simulink model "Currentreqtest"  (R2022a)
settings: Solver=FixedStepDiscrete  StartTime=0.0  StopTime=inf  FixedStep=0.01  RelTol=1e-3  EnableMultiTasking=on
libraries: mcp2515lib x32, simulink x29, svdutilitieslib x3, etargetslib x2
(part 1 of 2)
settings Model: Creator=Student  LastModifiedBy=Student
settings SolverCC: PositivePriorityOrder=on
settings OptimizationCC: EnhancedBackFolding=on  PassReuseOutputArgsAs=Individual arguments  ZeroExternalMemoryAtStartup=off  ZeroInternalMemoryAtStartup=off  MaxStackSize=64  OptimizeBlockOrder=speed  DifferentSizesBufferReuse=on  OptimizationCustomize=off  EfficientTunableParamExpr=on
settings DebuggingCC: ParameterTunabilityLossMsg=error
settings HardwareCC: ProdBitPerPointer=32  ProdBitPerSizeT=32  ProdBitPerPtrDiffT=32  ProdLargestAtomicInteger=Long  ProdLargestAtomicFloat=Double  ProdWordSize=32  ProdLongLongMode=on  ProdHWDeviceType=ARM Compatible->ARM Cortex  UseEmbeddedCoderFeatures=off
settings RTWCC: SystemTargetFile=ert.tlc  HardwareBoard=Raspberry Pi  TLCOptions="-aInlineSetEventsForThisBaseRateFcn=TLC_FALSE -aSuppressMultiTaskScheduler=TLC_FALSE  -aRateBasedStepFcn=0"  TemplateMakefile=ert_default_tmf  Toolchain=GNU GCC Embedded Linux  BuildConfiguration=Faster Runs
settings CodeAppCC: ForceParamTrailComments=on  IgnoreCustomStorageClasses=off  OperatorAnnotations=on  SimulinkDataObjDesc=on  SFDataObjDesc=on  InsertBlockDesc=on
settings ERTTargetCC: SupportNonInlinedSFcns=on  SupportVariableSizeSignals=on  ExtModeTransport=2  ExtModeStaticAlloc=on  ExtModeMexFile=ext_xcp  ExtModeIntrfLevel=Level2 - Open

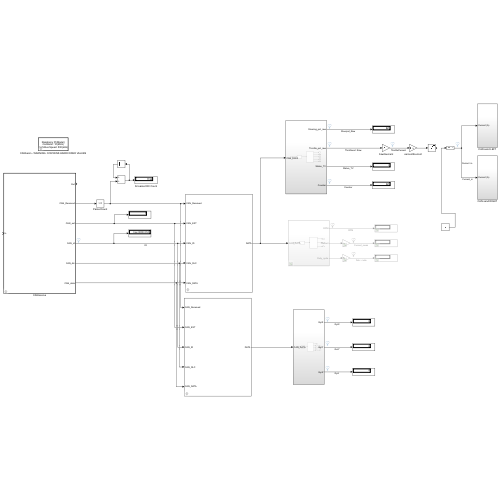
[thumbnail: Simulink's stored preview of the top-level diagram]
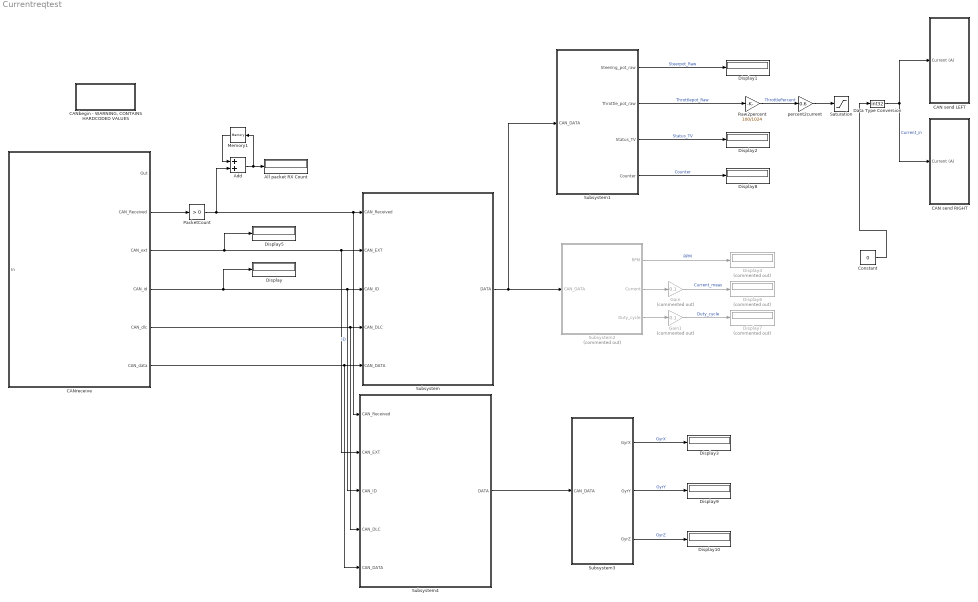
== system Currentreqtest ==
  Add : Sum  OutDataTypeStr=uint32
  All packet RX Count : Display
  CAN send LEFT : Subsystem
  CAN send RIGHT : Subsystem
  "CANbegin - WARNING, CONTAINS HARDCODED VALUES" : Subsystem  TreatAsAtomicUnit=on  mask{TargetHardware=Raspberry Pi, Oscillator=10, CANSpeed=500, CSpin=10}
      mask prompts: TargetHardware "Target Hardware"; Oscillator "Oscillator frequency(MHz)"; CANSpeed "CAN speed(kHz)"; CSpin "Chip Select Pin"
      mask init:
      | % Get this mask's handle
      | maskObj = Simulink.Mask.get(gcb);
      | 
      | % Get the selected value from mask parameter's option
      | str_TargetHard = char(maskObj.Parameters(1).TypeOptions(TargetHardware));
      | str_Osc = char(maskObj.Parameters(2).TypeOptions(Oscillator));
      | str_CANSpeed = char(maskObj.Parameters(3).TypeOptions(CANSpeed));
      | 
      | % Set Icon
      | str1 = sprintf('%s(Model)',str_TargetHard);
      | str2 = sprintf('Oscillator: %s(MHz)',str_Osc);
      | str3 = sprintf('CAN Bus Speed: %s(kHz)',str_CANSpeed);
      | str4 = sprintf('Chip Select pin: %d',CSpin);
      | 
      | % Set the values of Variant Subsystem
      | switch str_TargetHard
      |     case 'Arduino'
      |         str = [str1,'\n',str2,'\n',str3,'\n',str4];
      |         evalin('base',sprintf('CSpin = %d;',CSpin));        
      |         evalin('base','Hardware = 1;');
      |     case 'Raspberry Pi'
      |         str = [str1,'\n',str2,'\n',str3];
      |         evalin('base',sprintf('clear CSpin',CSpin));           
      |         evalin('base','Hardware = 2;');     
      | end  
      | 
      | % Get the CAN Configuration register's value from mask parameter's option
      | if str_Osc == '8' %[MHz]
      |     switch str_CANSpeed
      |         case '1000'
      |             BPR = 0; PHSEG1 = 0; PRSEG = 0; PHSEG2 = 0;
      |         case '500'
      |             BPR = 0; PHSEG1 = 2; PRSEG = 0; PHSEG2 = 2;
      |         case '250'
      |             BPR = 0; PHSEG1 = 6; PRSEG = 0; PHSEG2 = 6;
      |         case '125'
      |             BPR = 1; PHSEG1 = 6; PRSEG = 1; PHSEG2 = 5;
      |         case '100'
      |             BPR = 1; PHSEG1 = 7; PRSEG = 2; PHSEG2 = 7;
      |         case '83.3'
      |             BPR = 1; PHSEG1 = 7; PRSEG = 6; PHSEG2 = 7;
      |         case '62.5'
      |             BPR = 3; PHSEG1 = 6; PRSEG = 0; PHSEG2 = 6;
      |         case '50'
      |             BPR = 3; PHSEG1 = 7; PRSEG = 2; PHSEG2 = 7;
      |         case '33.3'
      |             BPR = 4; PHSEG1 = 7; PRSEG = 6; PHSEG2 = 7;
      |     end            
      | elseif str_Osc == '16' %[MHz]
      |     switch str_CANSpeed  
      |         case '1000'
      |             BPR = 0; PHSEG1 = 2; PRSEG = 0; PHSEG2 = 2;
      |         case '500'
      |             BPR = 0; PHSEG1 = 6; PRSEG = 0; PHSEG2 = 6;
      |         case '250'
      |             BPR = 1; PHSEG1 = 6; PRSEG = 1; PHSEG2 = 5;        
      |         case '125'
      |             BPR = 3; PHSEG1 = 6; PRSEG = 0; PHSEG2 = 6;
      |         case '100'
      |             BPR = 3; PHSEG1 = 7; PRSEG = 2; PHSEG2 = 7;
      |         case '83.3'
      |             BPR = 3; PHSEG1 = 7; PRSEG = 6; PHSEG2 = 7;
      |         case '62.5'
      |             BPR = 7; PHSEG1 = 6; PRSEG = 0; PHSEG2 = 6;
      |         case '50'
      |             BPR = 7; PHSEG1 = 7; PRSEG = 2; PHSEG2 = 7;
      |         case '33.3'
      |             BPR = 9; PHSEG1 = 7; PRSEG = 6; PHSEG2 = 7;        
      |     end
      |     
      | elseif str_Osc == '10' %[MHz]
      |     switch str_CANSpeed  
      |         case '1000'
      |             BPR = 0; PHSEG1 = 2; PRSEG = 0; PHSEG2 = 2;
      |         case '500'
      |             BPR = 0; PHSEG1 = 5; PRSEG = 0; PHSEG2 = 4;
      |         case '250'
      |             BPR = 1; PHSEG1 = 6; PRSEG = 1; PHSEG2 = 5;        
      |         case '125'
      |             BPR = 3; PHSEG1 = 6; PRSEG = 0; PHSEG2 = 6;
      |         case '100'
      |             BPR = 3; PHSEG1 = 7; PRSEG = 2; PHSEG2 = 7;
      |         case '83.3'
      |             BPR = 3; PHSEG1 = 7; PRSEG = 6; PHSEG2 = 7;
      |         case '62.5'
      |             BPR = 7; PHSEG1 = 6; PRSEG = 0; PHSEG2 = 6;
      |         case '50'
      |             BPR = 7; PHSEG1 = 7; PRSEG = 2; PHSEG2 = 7;
      |         case '33.3'
      |             BPR = 9; PHSEG1 = 7; PRSEG = 6; PHSEG2 = 7;        
      |     end    
      |     
      |     
      | end
      | % % Set the CAN Configuration register's value
      | % address2A = BPR;          % bit7-6 :SJW, bit5-0: BPR
      | % address29 = 192 ...       % bit7: BTLMODE = 1, bit6:SAM = 1
      | %             + 8*PHSEG1 ...% bit5-3: PHSEG1
      | %             +PRSEG;       % bit2-0: PRSEG
      | % address28 = 128 ...       % bit7: SOF = 1, bit6:WAKFIL = 0
      | %             + PHSEG2;     % bit5-3: 0, bit2-0: PHSEG2
      |         
      | % force parameters... 
      | % %1M CAN
      | % address2A=hex2dec('40')
      | % address29=hex2dec('80')
      | % address28=hex2dec('1')
      | 
      | %500k CAN
      | address2A=hex2dec('0')
      | address29=hex2dec('A0')
      | address28=hex2dec('02')
      | 
      | % %500k CAN from Arduino library spreadsheet - doesn't work
      | % address2A=hex2dec('41')
      | % address29=hex2dec('D9')
      | % address28=hex2dec('82')
      settings: RTWSystemCode=Nonreusable function
      mask TypeOptions TargetHardware: Arduino | Raspberry Pi
      mask Callback TargetHardware:
      | if(strcmp(get_param(gcb,'TargetHardware'),'Arduino'))
      |     set_param(gcb,'MaskVisibilities',{'on','on','on','on'})
      | else
      |     set_param(gcb,'MaskVisibilities',{'on','on','on','off'})
      | end
      mask TypeOptions Oscillator: 8 | 16 | 10
      mask TypeOptions CANSpeed: 1000 | 500 | 250 | 125 | 100 | 83.3 | 62.5 | 50 | 33.3
      mask DialogControl DescGroupVar Prompt: Description
      mask DialogControl DescTextVar Prompt: Forced parameters for 10MHz oscillator, 500k CAN This block must be executed only once when beginning CAN communication because MCP2515’s register needs to be configured. And the frequency of oscillator for MCP2515 is also needed because it effects to the setting parameters of MCP2515's register.
      mask Display: disp(str)
  CANreceive : Subsystem  TreatAsAtomicUnit=on
      mask DialogControl DescGroupVar Prompt: Description
      mask DialogControl DescTextVar Prompt: CANreceive outputs CAN data by converting MCP2515 RX buffer register’s values. In/Out ports are no use because they are used for controlling the execution order. CAN_Received outputs 1(CAN received) or -1( No message).
  Constant : Constant  Value=0
  Data Type Conversion : DataTypeConversion  OutDataTypeStr=int32  SaturateOnIntegerOverflow=off  RndMeth=Floor
  Display{,1..3,5,8..10} (8 alike) : Display
      Display settings: Format=hex (Stored Integer)
  Display4 : Display  Commented=on
  Display6 : Display  Commented=on
  Display7 : Display  Commented=on
  Gain : Gain  Commented=on  Gain=0.1
  Gain1 : Gain  Commented=on  Gain=0.1
  Memory1 : Memory  InitialCondition=[0]
  "PacketCount " : simulink/Logic and Bit Operations/Compare To Constant  relop=>  const=0  OutDataTypeStr=uint8
  Raw2percent : Gain  Gain=100/1024
  Saturation : Saturate  UpperLimit=40  LowerLimit=0
  Subsystem : Subsystem  mask{ID=0x123, DLC=6, EXT=1}
      mask prompts: ID "Message ID"; DLC "Message DLC"; EXT "Type of ID (1 is extended, 0 is standard)"
      mask DialogControl DescGroupVar Prompt: Filter CAN Data
      mask DialogControl DescTextVar Prompt: Give the ID and DLC of the CAN Message you want to get the data from
  Subsystem1 : Subsystem
  Subsystem2 : Subsystem  Commented=on
  Subsystem3 : Subsystem
  Subsystem4 : Subsystem  mask{ID=0x32, DLC=6, EXT=1}
      mask prompts: ID "Message ID"; DLC "Message DLC"; EXT "Type of ID (1 is extended, 0 is standard)"
      mask DialogControl DescGroupVar Prompt: Filter CAN Data
      mask DialogControl DescTextVar Prompt: Give the ID and DLC of the CAN Message you want to get the data from
  percent2current : Gain  Gain=0.6
  wires:
  Gain1/1 -> Display7/1  "Duty_cycle"
  "PacketCount "/1 -> Add/2, Subsystem4/1(CAN_Received), Subsystem/1(CAN_Received)
  Memory1/1 -> Add/1
  Subsystem2/3(Duty_cycle) -> Gain1/1
  Gain/1 -> Display6/1  "Current_meas"
  Subsystem2/1(RPM) -> Display4/1  "RPM"
  Subsystem1/1(Steering_pot_raw) -> Display1/1  "Steerpot_Raw"
  CANreceive/5(CAN_dlc) -> Subsystem/4(CAN_DLC), Subsystem4/4(CAN_DLC)
  Subsystem2/2(Current) -> Gain/1
  Subsystem1/3(Status_TV) -> Display2/1  "Status_TV"
  Subsystem1/2(Throttle_pot_raw) -> Raw2percent/1  "Throttlepot_Raw"
  CANreceive/4(CAN_id) -> Display/1, Subsystem/3(CAN_ID), Subsystem4/3(CAN_ID)  "ID"
  Add/1 -> All packet RX Count/1, Memory1/1
  Subsystem/1(DATA) -> Subsystem1/1(CAN_DATA), Subsystem2/1(CAN_DATA)
  CANreceive/3(CAN_ext) -> Display5/1, Subsystem/2(CAN_EXT), Subsystem4/2(CAN_EXT)
  CANreceive/2(CAN_Received) -> "PacketCount "/1
  CANreceive/6(CAN_data) -> Subsystem/5(CAN_DATA), Subsystem4/5(CAN_DATA)
  Data Type Conversion/1 -> CAN send RIGHT/1(Current (A)), CAN send LEFT/1(Current (A))  "Current_in"
  Subsystem1/4(Counter) -> Display8/1  "Counter"
  Raw2percent/1 -> percent2current/1  "ThrottlePercent"
  percent2current/1 -> Saturation/1
  Subsystem3/1(GyrX) -> Display3/1  "GyrX"
  Subsystem3/2(GyrY) -> Display9/1  "GyrY"
  Subsystem3/3(GyrZ) -> Display10/1  "GyrZ"
  Subsystem4/1(DATA) -> Subsystem3/1(CAN_DATA)
  Constant/1 -> Data Type Conversion/1

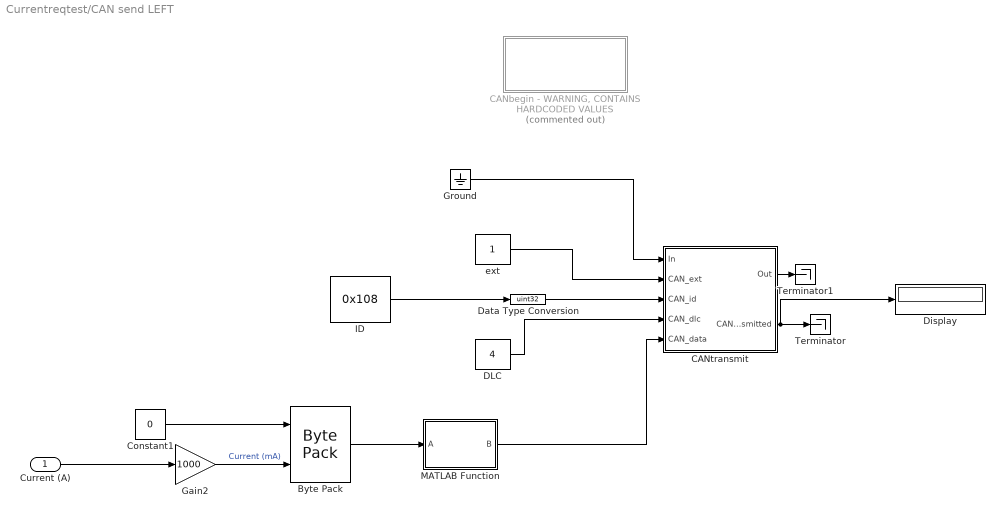
== system Currentreqtest/CAN send LEFT ==
  Current (A) : Inport  OutDataTypeStr=int32
  Byte Pack : etargetslib/Byte Pack  datatypes={'int32','int32'}  byteAlign=1
  "CANbegin - WARNING, CONTAINS HARDCODED VALUES" : Subsystem  Commented=on  TreatAsAtomicUnit=on  mask{TargetHardware=Raspberry Pi, Oscillator=10, CANSpeed=500, CSpin=10}
      mask prompts: TargetHardware "Target Hardware"; Oscillator "Oscillator frequency(MHz)"; CANSpeed "CAN speed(kHz)"; CSpin "Chip Select Pin"
      mask init: same as Currentreqtest/CANbegin - WARNING, CONTAINS HARDCODED VALUES
      settings: RTWSystemCode=Nonreusable function
      mask TypeOptions TargetHardware: Arduino | Raspberry Pi
      mask Callback TargetHardware:
      | if(strcmp(get_param(gcb,'TargetHardware'),'Arduino'))
      |     set_param(gcb,'MaskVisibilities',{'on','on','on','on'})
      | else
      |     set_param(gcb,'MaskVisibilities',{'on','on','on','off'})
      | end
      mask TypeOptions Oscillator: 8 | 16 | 10
      mask TypeOptions CANSpeed: 1000 | 500 | 250 | 125 | 100 | 83.3 | 62.5 | 50 | 33.3
      mask DialogControl DescGroupVar Prompt: Description
      mask DialogControl DescTextVar Prompt: Forced parameters for 10MHz oscillator, 500k CAN This block must be executed only once when beginning CAN communication because MCP2515’s register needs to be configured. And the frequency of oscillator for MCP2515 is also needed because it effects to the setting parameters of MCP2515's register.
      mask Display: disp(str)
  CANtransmit : Subsystem  TreatAsAtomicUnit=on
      mask DialogControl DescGroupVar Prompt: Description
      mask DialogControl DescTextVar Prompt: CANtransmit inputs CAN data by converting MCP2515 TX buffer register’s values. In/Out ports are no use because they are used for controlling the execution order. CAN_Transmitted outputs 1(Success) or 2(Fail).
  Constant1 : Constant  Value=0  OutDataTypeStr=int32
  DLC : Constant  Value=4  OutDataTypeStr=uint8
  Data Type Conversion : DataTypeConversion  OutDataTypeStr=uint32  SaturateOnIntegerOverflow=off  RndMeth=Floor
  Display : Display
  Gain2 : Gain  Gain=1000  OutDataTypeStr=int32
  Ground : Ground
  ID : Constant  Value=0x108  OutDataTypeStr=uint32
  MATLAB Function : MATLAB Function  TreatAsAtomicUnit=on
  Terminator : Terminator
  Terminator1 : Terminator
  ext : Constant  OutDataTypeStr=uint8
  wires:
  Byte Pack/1 -> MATLAB Function/1(A)
  Ground/1 -> CANtransmit/1(In)
  ext/1 -> CANtransmit/2(CAN_ext)
  DLC/1 -> CANtransmit/4(CAN_dlc)
  CANtransmit/1(Out) -> Terminator1/1
  CANtransmit/2(CAN_Transmitted) -> Display/1, Terminator/1
  Data Type Conversion/1 -> CANtransmit/3(CAN_id)
  Constant1/1 -> Byte Pack/1
  MATLAB Function/1(B) -> CANtransmit/5(CAN_data)
  Current (A)/1 -> Gain2/1
  Gain2/1 -> Byte Pack/2  "Current (mA)"
  ID/1 -> Data Type Conversion/1

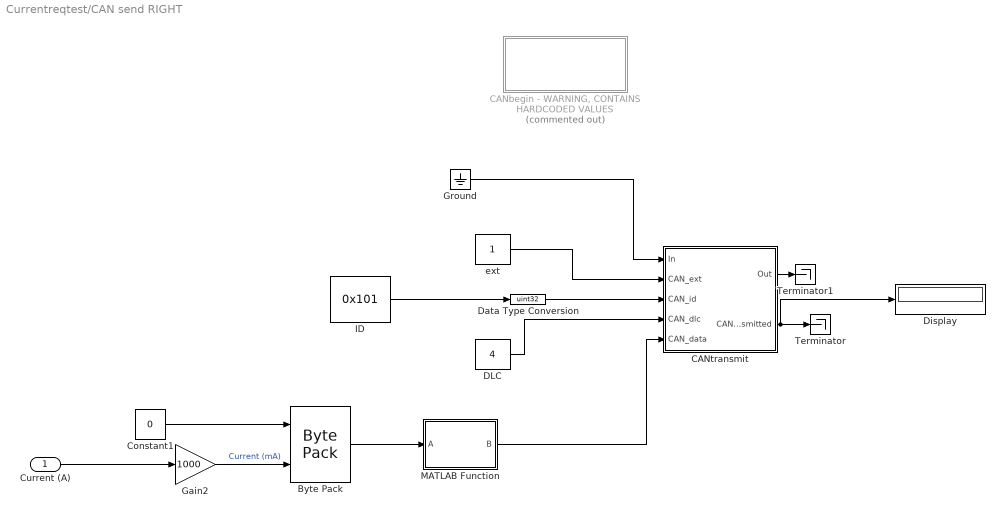
== system Currentreqtest/CAN send RIGHT ==
  Current (A) : Inport  OutDataTypeStr=int32
  Byte Pack : etargetslib/Byte Pack  datatypes={'int32','int32'}  byteAlign=1
  "CANbegin - WARNING, CONTAINS HARDCODED VALUES" : Subsystem  Commented=on  TreatAsAtomicUnit=on  mask{TargetHardware=Raspberry Pi, Oscillator=10, CANSpeed=500, CSpin=10}
      mask prompts: TargetHardware "Target Hardware"; Oscillator "Oscillator frequency(MHz)"; CANSpeed "CAN speed(kHz)"; CSpin "Chip Select Pin"
      mask init: same as Currentreqtest/CANbegin - WARNING, CONTAINS HARDCODED VALUES
      settings: RTWSystemCode=Nonreusable function
      mask TypeOptions TargetHardware: Arduino | Raspberry Pi
      mask Callback TargetHardware:
      | if(strcmp(get_param(gcb,'TargetHardware'),'Arduino'))
      |     set_param(gcb,'MaskVisibilities',{'on','on','on','on'})
      | else
      |     set_param(gcb,'MaskVisibilities',{'on','on','on','off'})
      | end
      mask TypeOptions Oscillator: 8 | 16 | 10
      mask TypeOptions CANSpeed: 1000 | 500 | 250 | 125 | 100 | 83.3 | 62.5 | 50 | 33.3
      mask DialogControl DescGroupVar Prompt: Description
      mask DialogControl DescTextVar Prompt: Forced parameters for 10MHz oscillator, 500k CAN This block must be executed only once when beginning CAN communication because MCP2515’s register needs to be configured. And the frequency of oscillator for MCP2515 is also needed because it effects to the setting parameters of MCP2515's register.
      mask Display: disp(str)
  CANtransmit : Subsystem  TreatAsAtomicUnit=on
      mask DialogControl DescGroupVar Prompt: Description
      mask DialogControl DescTextVar Prompt: CANtransmit inputs CAN data by converting MCP2515 TX buffer register’s values. In/Out ports are no use because they are used for controlling the execution order. CAN_Transmitted outputs 1(Success) or 2(Fail).
  Constant1 : Constant  Value=0  OutDataTypeStr=int32
  DLC : Constant  Value=4  OutDataTypeStr=uint8
  Data Type Conversion : DataTypeConversion  OutDataTypeStr=uint32  SaturateOnIntegerOverflow=off  RndMeth=Floor
  Display : Display
  Gain2 : Gain  Gain=1000  OutDataTypeStr=int32
  Ground : Ground
  ID : Constant  Value=0x101  OutDataTypeStr=uint32
  MATLAB Function : MATLAB Function  TreatAsAtomicUnit=on
  Terminator : Terminator
  Terminator1 : Terminator
  ext : Constant  OutDataTypeStr=uint8
  wires:
  Byte Pack/1 -> MATLAB Function/1(A)
  Ground/1 -> CANtransmit/1(In)
  ext/1 -> CANtransmit/2(CAN_ext)
  DLC/1 -> CANtransmit/4(CAN_dlc)
  CANtransmit/1(Out) -> Terminator1/1
  CANtransmit/2(CAN_Transmitted) -> Display/1, Terminator/1
  Data Type Conversion/1 -> CANtransmit/3(CAN_id)
  Constant1/1 -> Byte Pack/1
  MATLAB Function/1(B) -> CANtransmit/5(CAN_data)
  Current (A)/1 -> Gain2/1
  Gain2/1 -> Byte Pack/2  "Current (mA)"
  ID/1 -> Data Type Conversion/1

== system Currentreqtest/CANbegin - WARNING, CONTAINS HARDCODED VALUES ==
  Constant : Constant  Value=0  OutDataTypeStr=boolean  SampleTime=-1
  Temporary buffer : DataStoreMemory  DataStoreName=temp_1byte  ReadBeforeWriteMsg=warning  WriteAfterWriteMsg=warning  WriteAfterReadMsg=warning  ShowAdditionalParam=off  OutDataTypeStr=uint8
  Unit Delay : UnitDelay  InitialCondition=1  SampleTime=-1  HasFrameUpgradeWarning=on
  setup : Subsystem  TreatAsAtomicUnit=on
      settings: RTWSystemCode=Nonreusable function  RTWFileNameOpts=Use subsystem name
  wires:
  Unit Delay/1 -> setup/Enable
  Constant/1 -> Unit Delay/1

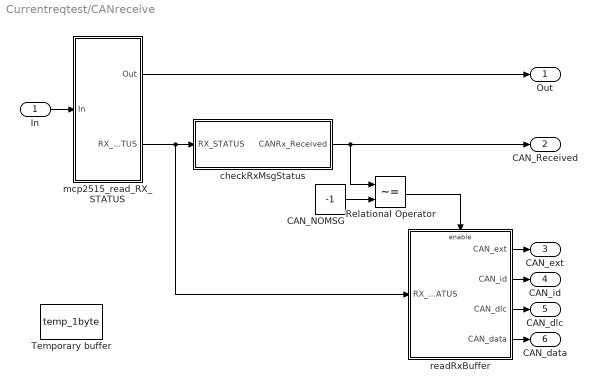
== system Currentreqtest/CANreceive ==
  In : Inport
  CAN_NOMSG : Constant  Value=-1  OutDataTypeStr=int8
  Relational Operator : RelationalOperator  Operator=~=  OutDataTypeStr=boolean  InputSameDT=off
  Temporary buffer : DataStoreMemory  DataStoreName=temp_1byte  ReadBeforeWriteMsg=warning  WriteAfterWriteMsg=warning  WriteAfterReadMsg=warning  ShowAdditionalParam=off  OutDataTypeStr=uint8
  checkRxMsgStatus : Subsystem  TreatAsAtomicUnit=on
  mcp2515_read_RX_STATUS : Subsystem  TreatAsAtomicUnit=on
  readRxBuffer : Subsystem  TreatAsAtomicUnit=on
  Out : Outport
  CAN_Received : Outport  Port=2
  CAN_ext : Outport  Port=3
  CAN_id : Outport  Port=4
  CAN_dlc : Outport  Port=5
  CAN_data : Outport  Port=6
  wires:
  In/1 -> mcp2515_read_RX_STATUS/1(In)
  mcp2515_read_RX_STATUS/1(Out) -> Out/1
  checkRxMsgStatus/1(CANRx_Received) -> CAN_Received/1, Relational Operator/1
  mcp2515_read_RX_STATUS/2(RX_STATUS) -> readRxBuffer/1(RX_STATUS), checkRxMsgStatus/1(RX_STATUS)
  readRxBuffer/1(CAN_ext) -> CAN_ext/1
  readRxBuffer/2(CAN_id) -> CAN_id/1
  readRxBuffer/3(CAN_dlc) -> CAN_dlc/1
  readRxBuffer/4(CAN_data) -> CAN_data/1
  CAN_NOMSG/1 -> Relational Operator/2
  Relational Operator/1 -> readRxBuffer/Enable

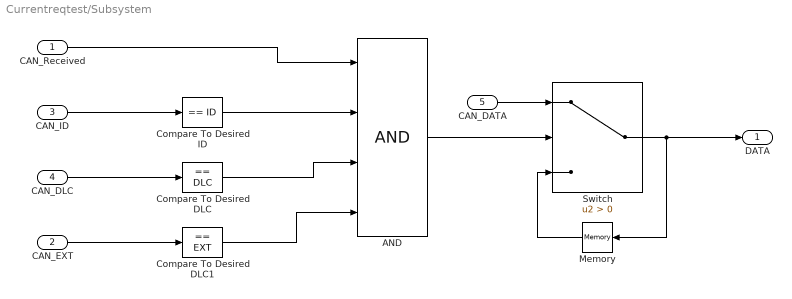
== system Currentreqtest/Subsystem ==
  CAN_Received : Inport
  CAN_EXT : Inport  Port=2
  CAN_ID : Inport  Port=3
  CAN_DLC : Inport  Port=4
  CAN_DATA : Inport  Port=5
  AND : Logic  Inputs=4  IconShape=distinctive  AllPortsSameDT=off  OutDataTypeStr=boolean
  Compare To Desired DLC : simulink/Logic and Bit Operations/Compare To Constant  relop===  const=DLC  OutDataTypeStr=boolean
  Compare To Desired DLC1 : simulink/Logic and Bit Operations/Compare To Constant  relop===  const=EXT  OutDataTypeStr=boolean
  Compare To Desired ID : simulink/Logic and Bit Operations/Compare To Constant  relop===  const=ID  OutDataTypeStr=boolean
  Memory : Memory
  Switch : Switch  Criteria=u2 > Threshold  SaturateOnIntegerOverflow=off  InputSameDT=off
  DATA : Outport
  wires:
  CAN_ID/1 -> Compare To Desired ID/1
  CAN_DLC/1 -> Compare To Desired DLC/1
  Compare To Desired DLC/1 -> AND/3
  Compare To Desired ID/1 -> AND/2
  CAN_Received/1 -> AND/1
  AND/1 -> Switch/2
  CAN_DATA/1 -> Switch/1
  Switch/1 -> DATA/1, Memory/1
  Memory/1 -> Switch/3
  CAN_EXT/1 -> Compare To Desired DLC1/1
  Compare To Desired DLC1/1 -> AND/4

== system Currentreqtest/Subsystem1 ==
  CAN_DATA : Inport
  Byte Unpack : svdutilitieslib/Byte Unpack  dimensions={[1], [1], [1], [1], [1]}  datatypes={['uint16'], ['uint8'], ['uint8'], ['uint16'], ['uint16']}  byteAlign=1  blockPlatform=arduinoert
      settings: SourceProductBaseCode=ANDROID,ARDUINO,ML_ARDUINO,ECCORTEXA,ECCORTEXR,SC_BEAGLEBONE_BLUE,EC_FREEDOM_BOARD,EC_FRDM_K64F,INTEL_BLOCKSET,MICROBIT,NUCLEO,NVIDIA,PX4AUTOPILOTS,RASPPIIO,STMICRODIS,TIC2000,XILINX_BLOCKSET
  MATLAB Function : MATLAB Function  TreatAsAtomicUnit=on
  Terminator : Terminator
  Steering_pot_raw : Outport
  Throttle_pot_raw : Outport  Port=2
  Status_TV : Outport  Port=3
  Counter : Outport  Port=4
  wires:
  CAN_DATA/1 -> MATLAB Function/1(A)
  MATLAB Function/1(B) -> Byte Unpack/1
  Byte Unpack/1 -> Terminator/1
  Byte Unpack/2 -> Counter/1
  Byte Unpack/4 -> Throttle_pot_raw/1
  Byte Unpack/5 -> Steering_pot_raw/1
  Byte Unpack/3 -> Status_TV/1

== system Currentreqtest/Subsystem2 ==
  CAN_DATA : Inport
  Byte Unpack : svdutilitieslib/Byte Unpack  dimensions={[1], [1], [1]}  datatypes={['int16'], ['int16'], ['int32']}  byteAlign=1  blockPlatform=arduinoert
      settings: SourceProductBaseCode=ANDROID,ARDUINO,ML_ARDUINO,ECCORTEXA,ECCORTEXR,SC_BEAGLEBONE_BLUE,EC_FREEDOM_BOARD,EC_FRDM_K64F,INTEL_BLOCKSET,MICROBIT,NUCLEO,NVIDIA,PX4AUTOPILOTS,RASPPIIO,STMICRODIS,TIC2000,XILINX_BLOCKSET
  MATLAB Function : MATLAB Function  TreatAsAtomicUnit=on
  RPM : Outport
  Current : Outport  Port=2
  Duty_cycle : Outport  Port=3
  wires:
  Byte Unpack/3 -> RPM/1
  Byte Unpack/1 -> Duty_cycle/1
  CAN_DATA/1 -> MATLAB Function/1(A)
  Byte Unpack/2 -> Current/1
  MATLAB Function/1(B) -> Byte Unpack/1

== system Currentreqtest/Subsystem3 ==
  CAN_DATA : Inport
  Byte Unpack : svdutilitieslib/Byte Unpack  dimensions={[1], [1], [1], [1]}  datatypes="{['int16'],  ['int16'], ['int16'], ['int16']}"  byteAlign=1  blockPlatform=arduinoert
      settings: SourceProductBaseCode=ANDROID,ARDUINO,ML_ARDUINO,ECCORTEXA,ECCORTEXR,SC_BEAGLEBONE_BLUE,EC_FREEDOM_BOARD,EC_FRDM_K64F,INTEL_BLOCKSET,MICROBIT,NUCLEO,NVIDIA,PX4AUTOPILOTS,RASPPIIO,STMICRODIS,TIC2000,XILINX_BLOCKSET
  MATLAB Function : MATLAB Function  TreatAsAtomicUnit=on
  Raw2phys : Gain  Gain=2^(-9)
  Raw2phys1 : Gain  Gain=2^(-9)
  Raw2phys2 : Gain  Gain=2^(-9)
  Terminator : Terminator
  GyrX : Outport
  GyrY : Outport  Port=2
  GyrZ : Outport  Port=3
  wires:
  CAN_DATA/1 -> MATLAB Function/1(A)
  MATLAB Function/1(B) -> Byte Unpack/1
  Byte Unpack/1 -> Terminator/1
  Byte Unpack/2 -> Raw2phys/1
  Byte Unpack/3 -> Raw2phys1/1
  Byte Unpack/4 -> Raw2phys2/1
  Raw2phys/1 -> GyrZ/1
  Raw2phys1/1 -> GyrY/1
  Raw2phys2/1 -> GyrX/1

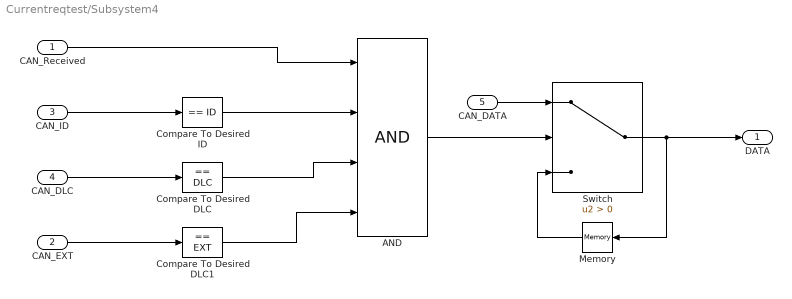
== system Currentreqtest/Subsystem4 ==
  CAN_Received : Inport
  CAN_EXT : Inport  Port=2
  CAN_ID : Inport  Port=3
  CAN_DLC : Inport  Port=4
  CAN_DATA : Inport  Port=5
  AND : Logic  Inputs=4  IconShape=distinctive  AllPortsSameDT=off  OutDataTypeStr=boolean
  Compare To Desired DLC : simulink/Logic and Bit Operations/Compare To Constant  relop===  const=DLC  OutDataTypeStr=boolean
  Compare To Desired DLC1 : simulink/Logic and Bit Operations/Compare To Constant  relop===  const=EXT  OutDataTypeStr=boolean
  Compare To Desired ID : simulink/Logic and Bit Operations/Compare To Constant  relop===  const=ID  OutDataTypeStr=boolean
  Memory : Memory
  Switch : Switch  Criteria=u2 > Threshold  SaturateOnIntegerOverflow=off  InputSameDT=off
  DATA : Outport
  wires:
  CAN_ID/1 -> Compare To Desired ID/1
  CAN_DLC/1 -> Compare To Desired DLC/1
  Compare To Desired DLC/1 -> AND/3
  Compare To Desired ID/1 -> AND/2
  CAN_Received/1 -> AND/1
  AND/1 -> Switch/2
  CAN_DATA/1 -> Switch/1
  Switch/1 -> DATA/1, Memory/1
  Memory/1 -> Switch/3
  CAN_EXT/1 -> Compare To Desired DLC1/1
  Compare To Desired DLC1/1 -> AND/4

== system Currentreqtest/CAN send LEFT/CANbegin - WARNING, CONTAINS HARDCODED VALUES ==
  Constant : Constant  Value=0  OutDataTypeStr=boolean  SampleTime=-1
  Temporary buffer : DataStoreMemory  DataStoreName=temp_1byte  ReadBeforeWriteMsg=warning  WriteAfterWriteMsg=warning  WriteAfterReadMsg=warning  ShowAdditionalParam=off  OutDataTypeStr=uint8
  Unit Delay : UnitDelay  InitialCondition=1  SampleTime=-1  HasFrameUpgradeWarning=on
  setup : Subsystem  TreatAsAtomicUnit=on
      settings: RTWSystemCode=Nonreusable function  RTWFileNameOpts=Use subsystem name
  wires:
  Unit Delay/1 -> setup/Enable
  Constant/1 -> Unit Delay/1

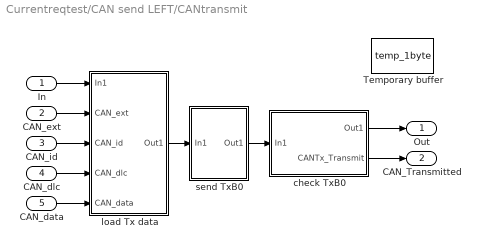
== system Currentreqtest/CAN send LEFT/CANtransmit ==
  In : Inport
  CAN_ext : Inport  Port=2
  CAN_id : Inport  Port=3
  CAN_dlc : Inport  Port=4
  CAN_data : Inport  Port=5
  Temporary buffer : DataStoreMemory  DataStoreName=temp_1byte  ReadBeforeWriteMsg=warning  WriteAfterWriteMsg=warning  WriteAfterReadMsg=warning  ShowAdditionalParam=off  OutDataTypeStr=uint8
  check TxB0 : Subsystem  TreatAsAtomicUnit=on
  load Tx data : Subsystem  TreatAsAtomicUnit=on
  send TxB0 : Subsystem  TreatAsAtomicUnit=on
  Out : Outport  VectorParamsAs1DForOutWhenUnconnected=off
  CAN_Transmitted : Outport  Port=2  VectorParamsAs1DForOutWhenUnconnected=off
  wires:
  In/1 -> load Tx data/1(In1)
  load Tx data/1(Out1) -> send TxB0/1(In1)
  send TxB0/1(Out1) -> check TxB0/1(In1)
  check TxB0/1(Out1) -> Out/1
  check TxB0/2(CANTx_Transmit) -> CAN_Transmitted/1
  CAN_ext/1 -> load Tx data/2(CAN_ext)
  CAN_id/1 -> load Tx data/3(CAN_id)
  CAN_dlc/1 -> load Tx data/4(CAN_dlc)
  CAN_data/1 -> load Tx data/5(CAN_data)

== system Currentreqtest/CAN send RIGHT/CANbegin - WARNING, CONTAINS HARDCODED VALUES ==
  Constant : Constant  Value=0  OutDataTypeStr=boolean  SampleTime=-1
  Temporary buffer : DataStoreMemory  DataStoreName=temp_1byte  ReadBeforeWriteMsg=warning  WriteAfterWriteMsg=warning  WriteAfterReadMsg=warning  ShowAdditionalParam=off  OutDataTypeStr=uint8
  Unit Delay : UnitDelay  InitialCondition=1  SampleTime=-1  HasFrameUpgradeWarning=on
  setup : Subsystem  TreatAsAtomicUnit=on
      settings: RTWSystemCode=Nonreusable function  RTWFileNameOpts=Use subsystem name
  wires:
  Unit Delay/1 -> setup/Enable
  Constant/1 -> Unit Delay/1

== system Currentreqtest/CAN send RIGHT/CANtransmit ==
  In : Inport
  CAN_ext : Inport  Port=2
  CAN_id : Inport  Port=3
  CAN_dlc : Inport  Port=4
  CAN_data : Inport  Port=5
  Temporary buffer : DataStoreMemory  DataStoreName=temp_1byte  ReadBeforeWriteMsg=warning  WriteAfterWriteMsg=warning  WriteAfterReadMsg=warning  ShowAdditionalParam=off  OutDataTypeStr=uint8
  check TxB0 : Subsystem  TreatAsAtomicUnit=on
  load Tx data : Subsystem  TreatAsAtomicUnit=on
  send TxB0 : Subsystem  TreatAsAtomicUnit=on
  Out : Outport  VectorParamsAs1DForOutWhenUnconnected=off
  CAN_Transmitted : Outport  Port=2  VectorParamsAs1DForOutWhenUnconnected=off
  wires:
  In/1 -> load Tx data/1(In1)
  load Tx data/1(Out1) -> send TxB0/1(In1)
  send TxB0/1(Out1) -> check TxB0/1(In1)
  check TxB0/1(Out1) -> Out/1
  check TxB0/2(CANTx_Transmit) -> CAN_Transmitted/1
  CAN_ext/1 -> load Tx data/2(CAN_ext)
  CAN_id/1 -> load Tx data/3(CAN_id)
  CAN_dlc/1 -> load Tx data/4(CAN_dlc)
  CAN_data/1 -> load Tx data/5(CAN_data)

== system Currentreqtest/CANbegin - WARNING, CONTAINS HARDCODED VALUES/setup ==
  Enable : EnablePort
  CNF1 : Constant  Value=address2A  OutDataTypeStr=uint8
  CNF2 : Constant  Value=address29  OutDataTypeStr=uint8
  CNF3 : Constant  Value=address28  OutDataTypeStr=uint8
  Ground : Ground
  Terminator : Terminator
  changeCANmode(config) : Subsystem  TreatAsAtomicUnit=on
  changeCANmode(normal) : Subsystem  TreatAsAtomicUnit=on
  mcp2515_reset : Subsystem  TreatAsAtomicUnit=on
  setCANRxBuffer : Subsystem  TreatAsAtomicUnit=on
  setCANspeed : Subsystem  TreatAsAtomicUnit=on
  wires:
  CNF3/1 -> setCANspeed/4(CNF3)
  CNF2/1 -> setCANspeed/3(CNF2)
  CNF1/1 -> setCANspeed/2(CNF1)
  mcp2515_reset/1(Out) -> changeCANmode(config)/1(In)
  changeCANmode(config)/1(Out) -> setCANspeed/1(In)
  setCANspeed/1(Out) -> setCANRxBuffer/1(In)
  setCANRxBuffer/1(Out) -> changeCANmode(normal)/1(In)
  Ground/1 -> mcp2515_reset/1(In)
  changeCANmode(normal)/1(Out) -> Terminator/1

== system Currentreqtest/CANreceive/checkRxMsgStatus ==
  RX_STATUS : Inport
  Bitmask_RxBn : simulink/Logic and Bit Operations/Bitwise Operator  logicop=AND  UseBitMask=on  BitMask=bin2dec('11000000')  BitMaskRealWorld=Stored Integer
  CAN_NOMSG : Constant  Value=-1  OutDataTypeStr=int8
  CAN_OK : Constant  OutDataTypeStr=int8
  Switch : Switch  Criteria=u2 > Threshold  SaturateOnIntegerOverflow=off  InputSameDT=off
  CANRx_Received : Outport
  wires:
  RX_STATUS/1 -> Bitmask_RxBn/1
  CAN_OK/1 -> Switch/1
  CAN_NOMSG/1 -> Switch/3
  Switch/1 -> CANRx_Received/1
  Bitmask_RxBn/1 -> Switch/2

== system Currentreqtest/CANreceive/mcp2515_read_RX_STATUS ==
  In : Inport
  Constant : Constant  Value=0  OutDataTypeStr=uint8
  MCP_RX_STATUS : Constant  Value=hex2dec('B0')  OutDataTypeStr=uint8
  SPI driver : mcp2515lib/CAN application/mcp2515 driver/SPI driver  SystemSampleTime=-1  VariantActivationTime=update diagram  Latency=0  AutoFrameSizeCalculation=off
      settings: SourceProductName=CAN device driver for mcp2515
  Selector : Selector  IndexMode=Zero-based  InputPortWidth=2  IndexOptions=Index vector (dialog)  Indices=1  OutputSizes=1
  Vector Concatenate : Concatenate
  Out : Outport
  RX_STATUS : Outport  Port=2
  wires:
  In/1 -> Out/1
  Constant/1 -> Vector Concatenate/2
  SPI driver/1 -> Selector/1  "SPIstatus_ext_id"
  Selector/1 -> RX_STATUS/1
  MCP_RX_STATUS/1 -> Vector Concatenate/1
  Vector Concatenate/1 -> SPI driver/1

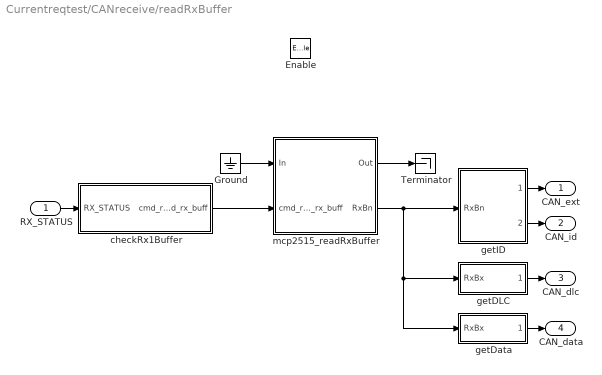
== system Currentreqtest/CANreceive/readRxBuffer ==
  RX_STATUS : Inport
  Enable : EnablePort
  Ground : Ground
  Terminator : Terminator
  checkRx1Buffer : Subsystem  TreatAsAtomicUnit=on
  getDLC : Subsystem  TreatAsAtomicUnit=on
  getData : Subsystem  TreatAsAtomicUnit=on
  getID : Subsystem  TreatAsAtomicUnit=on
      settings: RTWSystemCode=Inline
  mcp2515_readRxBuffer : Subsystem  TreatAsAtomicUnit=on
  CAN_ext : Outport
  CAN_id : Outport  Port=2
  CAN_dlc : Outport  Port=3
  CAN_data : Outport  Port=4
  wires:
  getData/1(CAN_data) -> CAN_data/1
  mcp2515_readRxBuffer/2(RxBn) -> getID/1(RxBn), getData/1(RxBx), getDLC/1(RxBx)
  getID/2(CAN_id) -> CAN_id/1
  getID/1(CAN_ext) -> CAN_ext/1
  getDLC/1(CAN_dlc) -> CAN_dlc/1
  mcp2515_readRxBuffer/1(Out) -> Terminator/1
  Ground/1 -> mcp2515_readRxBuffer/1(In)
  RX_STATUS/1 -> checkRx1Buffer/1(RX_STATUS)
  checkRx1Buffer/1(cmd_read_rx_buff) -> mcp2515_readRxBuffer/2(cmd_read_rx_buff)

== system Currentreqtest/CAN send LEFT/CANbegin - WARNING, CONTAINS HARDCODED VALUES/setup ==
  Enable : EnablePort
  CNF1 : Constant  Value=address2A  OutDataTypeStr=uint8
  CNF2 : Constant  Value=address29  OutDataTypeStr=uint8
  CNF3 : Constant  Value=address28  OutDataTypeStr=uint8
  Ground : Ground
  Terminator : Terminator
  changeCANmode(config) : Subsystem  TreatAsAtomicUnit=on
  changeCANmode(normal) : Subsystem  TreatAsAtomicUnit=on
  mcp2515_reset : Subsystem  TreatAsAtomicUnit=on
  setCANRxBuffer : Subsystem  TreatAsAtomicUnit=on
  setCANspeed : Subsystem  TreatAsAtomicUnit=on
  wires:
  CNF3/1 -> setCANspeed/4(CNF3)
  CNF2/1 -> setCANspeed/3(CNF2)
  CNF1/1 -> setCANspeed/2(CNF1)
  mcp2515_reset/1(Out) -> changeCANmode(config)/1(In)
  changeCANmode(config)/1(Out) -> setCANspeed/1(In)
  setCANspeed/1(Out) -> setCANRxBuffer/1(In)
  setCANRxBuffer/1(Out) -> changeCANmode(normal)/1(In)
  Ground/1 -> mcp2515_reset/1(In)
  changeCANmode(normal)/1(Out) -> Terminator/1

== system Currentreqtest/CAN send LEFT/CANtransmit/check TxB0 ==
  In1 : Inport
  Bitmask_TxReq : simulink/Logic and Bit Operations/Bitwise Operator  logicop=AND  UseBitMask=on  BitMask=bin2dec('00001000')  BitMaskRealWorld=Stored Integer
  CAN_FAIL : Constant  Value=2  OutDataTypeStr=int8
  CAN_OK : Constant  OutDataTypeStr=int8
  MCP_TxB0CTRL1 : Constant  Value=hex2dec('30')  OutDataTypeStr=uint8
  Switch : Switch  Criteria=u2 > Threshold  SaturateOnIntegerOverflow=off  InputSameDT=off
  mcp2515_readRegister : Subsystem  TreatAsAtomicUnit=on
  Out1 : Outport  VectorParamsAs1DForOutWhenUnconnected=off
  CANTx_Transmit : Outport  Port=2  VectorParamsAs1DForOutWhenUnconnected=off
  wires:
  CAN_FAIL/1 -> Switch/3
  mcp2515_readRegister/1(Out) -> Out1/1
  mcp2515_readRegister/2(SPI_data) -> Bitmask_TxReq/1
  MCP_TxB0CTRL1/1 -> mcp2515_readRegister/2(address)
  Bitmask_TxReq/1 -> Switch/2
  Switch/1 -> CANTx_Transmit/1
  CAN_OK/1 -> Switch/1
  In1/1 -> mcp2515_readRegister/1(In)

== system Currentreqtest/CAN send LEFT/CANtransmit/load Tx data ==
  In1 : Inport
  CAN_ext : Inport  Port=2
  CAN_id : Inport  Port=3
  CAN_dlc : Inport  Port=4
  CAN_data : Inport  Port=5
  MCP_load_TxB0 : Constant  Value=hex2dec('40')  OutDataTypeStr=uint8
  Vector Concatenate : Concatenate  NumInputs=3
  mcp2515_writeTxBuffer : Subsystem  TreatAsAtomicUnit=on
  setID : Subsystem  TreatAsAtomicUnit=on
      settings: RTWSystemCode=Inline
  Out1 : Outport  VectorParamsAs1DForOutWhenUnconnected=off
  wires:
  CAN_ext/1 -> setID/1(ext)
  CAN_id/1 -> setID/2(id)
  CAN_data/1 -> Vector Concatenate/3
  CAN_dlc/1 -> Vector Concatenate/2
  setID/1(TxBn_ID) -> Vector Concatenate/1
  In1/1 -> mcp2515_writeTxBuffer/1(In)
  mcp2515_writeTxBuffer/1(Out) -> Out1/1
  MCP_load_TxB0/1 -> mcp2515_writeTxBuffer/2(cmd_load_tx_buff)
  Vector Concatenate/1 -> mcp2515_writeTxBuffer/3(data_tx_buff)

== system Currentreqtest/CAN send LEFT/CANtransmit/send TxB0 ==
  In1 : Inport
  MCP_TxB0CTRL : Constant  Value=hex2dec('30')  OutDataTypeStr=uint8
  TxREQ : Constant  Value=8  OutDataTypeStr=uint8
  mcp2515_writeRegister : Subsystem  TreatAsAtomicUnit=on
  Out1 : Outport  VectorParamsAs1DForOutWhenUnconnected=off
  wires:
  MCP_TxB0CTRL/1 -> mcp2515_writeRegister/2(address)
  mcp2515_writeRegister/1(Out) -> Out1/1
  In1/1 -> mcp2515_writeRegister/1(In)
  TxREQ/1 -> mcp2515_writeRegister/3(value)

== system Currentreqtest/CAN send RIGHT/CANbegin - WARNING, CONTAINS HARDCODED VALUES/setup ==
  Enable : EnablePort
  CNF1 : Constant  Value=address2A  OutDataTypeStr=uint8
  CNF2 : Constant  Value=address29  OutDataTypeStr=uint8
  CNF3 : Constant  Value=address28  OutDataTypeStr=uint8
  Ground : Ground
  Terminator : Terminator
  changeCANmode(config) : Subsystem  TreatAsAtomicUnit=on
  changeCANmode(normal) : Subsystem  TreatAsAtomicUnit=on
  mcp2515_reset : Subsystem  TreatAsAtomicUnit=on
  setCANRxBuffer : Subsystem  TreatAsAtomicUnit=on
  setCANspeed : Subsystem  TreatAsAtomicUnit=on
  wires:
  CNF3/1 -> setCANspeed/4(CNF3)
  CNF2/1 -> setCANspeed/3(CNF2)
  CNF1/1 -> setCANspeed/2(CNF1)
  mcp2515_reset/1(Out) -> changeCANmode(config)/1(In)
  changeCANmode(config)/1(Out) -> setCANspeed/1(In)
  setCANspeed/1(Out) -> setCANRxBuffer/1(In)
  setCANRxBuffer/1(Out) -> changeCANmode(normal)/1(In)
  Ground/1 -> mcp2515_reset/1(In)
  changeCANmode(normal)/1(Out) -> Terminator/1

== system Currentreqtest/CAN send RIGHT/CANtransmit/check TxB0 ==
  In1 : Inport
  Bitmask_TxReq : simulink/Logic and Bit Operations/Bitwise Operator  logicop=AND  UseBitMask=on  BitMask=bin2dec('00001000')  BitMaskRealWorld=Stored Integer
  CAN_FAIL : Constant  Value=2  OutDataTypeStr=int8
  CAN_OK : Constant  OutDataTypeStr=int8
  MCP_TxB0CTRL1 : Constant  Value=hex2dec('30')  OutDataTypeStr=uint8
  Switch : Switch  Criteria=u2 > Threshold  SaturateOnIntegerOverflow=off  InputSameDT=off
  mcp2515_readRegister : Subsystem  TreatAsAtomicUnit=on
  Out1 : Outport  VectorParamsAs1DForOutWhenUnconnected=off
  CANTx_Transmit : Outport  Port=2  VectorParamsAs1DForOutWhenUnconnected=off
  wires:
  CAN_FAIL/1 -> Switch/3
  mcp2515_readRegister/1(Out) -> Out1/1
  mcp2515_readRegister/2(SPI_data) -> Bitmask_TxReq/1
  MCP_TxB0CTRL1/1 -> mcp2515_readRegister/2(address)
  Bitmask_TxReq/1 -> Switch/2
  Switch/1 -> CANTx_Transmit/1
  CAN_OK/1 -> Switch/1
  In1/1 -> mcp2515_readRegister/1(In)

== system Currentreqtest/CAN send RIGHT/CANtransmit/load Tx data ==
  In1 : Inport
  CAN_ext : Inport  Port=2
  CAN_id : Inport  Port=3
  CAN_dlc : Inport  Port=4
  CAN_data : Inport  Port=5
  MCP_load_TxB0 : Constant  Value=hex2dec('40')  OutDataTypeStr=uint8
  Vector Concatenate : Concatenate  NumInputs=3
  mcp2515_writeTxBuffer : Subsystem  TreatAsAtomicUnit=on
  setID : Subsystem  TreatAsAtomicUnit=on
      settings: RTWSystemCode=Inline
  Out1 : Outport  VectorParamsAs1DForOutWhenUnconnected=off
  wires:
  CAN_ext/1 -> setID/1(ext)
  CAN_id/1 -> setID/2(id)
  CAN_data/1 -> Vector Concatenate/3
  CAN_dlc/1 -> Vector Concatenate/2
  setID/1(TxBn_ID) -> Vector Concatenate/1
  In1/1 -> mcp2515_writeTxBuffer/1(In)
  mcp2515_writeTxBuffer/1(Out) -> Out1/1
  MCP_load_TxB0/1 -> mcp2515_writeTxBuffer/2(cmd_load_tx_buff)
  Vector Concatenate/1 -> mcp2515_writeTxBuffer/3(data_tx_buff)

== system Currentreqtest/CAN send RIGHT/CANtransmit/send TxB0 ==
  In1 : Inport
  MCP_TxB0CTRL : Constant  Value=hex2dec('30')  OutDataTypeStr=uint8
  TxREQ : Constant  Value=8  OutDataTypeStr=uint8
  mcp2515_writeRegister : Subsystem  TreatAsAtomicUnit=on
  Out1 : Outport  VectorParamsAs1DForOutWhenUnconnected=off
  wires:
  MCP_TxB0CTRL/1 -> mcp2515_writeRegister/2(address)
  mcp2515_writeRegister/1(Out) -> Out1/1
  In1/1 -> mcp2515_writeRegister/1(In)
  TxREQ/1 -> mcp2515_writeRegister/3(value)

== system Currentreqtest/CANbegin - WARNING, CONTAINS HARDCODED VALUES/setup/changeCANmode(config) ==
  In : Inport
  MCP_CANCTRL : Constant  Value=hex2dec('0F')  OutDataTypeStr=uint8
  MODE_CONFIG : Constant  Value=hex2dec('80')  OutDataTypeStr=uint8
  MODE_MASK : Constant  Value=hex2dec('E0')  OutDataTypeStr=uint8
  mcp2515_modifyRegister : Subsystem  TreatAsAtomicUnit=on
  Out : Outport  VectorParamsAs1DForOutWhenUnconnected=off
  wires:
  MODE_CONFIG/1 -> mcp2515_modifyRegister/4(data)
  MODE_MASK/1 -> mcp2515_modifyRegister/3(mask)
  MCP_CANCTRL/1 -> mcp2515_modifyRegister/2(address)
  In/1 -> mcp2515_modifyRegister/1(In)
  mcp2515_modifyRegister/1(Out) -> Out/1

== system Currentreqtest/CANbegin - WARNING, CONTAINS HARDCODED VALUES/setup/changeCANmode(normal) ==
  In : Inport
  MCP_CANCTRL : Constant  Value=hex2dec('0F')  OutDataTypeStr=uint8
  MODE_MASK : Constant  Value=hex2dec('E0')  OutDataTypeStr=uint8
  MODE_NORMAL : Constant  Value=0  OutDataTypeStr=uint8
  mcp2515_modifyRegister : Subsystem  TreatAsAtomicUnit=on
  Out : Outport  VectorParamsAs1DForOutWhenUnconnected=off
  wires:
  MODE_MASK/1 -> mcp2515_modifyRegister/3(mask)
  MODE_NORMAL/1 -> mcp2515_modifyRegister/4(data)
  MCP_CANCTRL/1 -> mcp2515_modifyRegister/2(address)
  In/1 -> mcp2515_modifyRegister/1(In)
  mcp2515_modifyRegister/1(Out) -> Out/1

== system Currentreqtest/CANbegin - WARNING, CONTAINS HARDCODED VALUES/setup/mcp2515_reset ==
  In : Inport
  MCP_RESET : Constant  Value=hex2dec('C0')  OutDataTypeStr=uint8
  SPI driver : mcp2515lib/CAN application/mcp2515 driver/SPI driver  SystemSampleTime=-1  VariantActivationTime=update diagram  Latency=0  AutoFrameSizeCalculation=off
      settings: SourceProductName=CAN device driver for mcp2515
  Temporary buffer : DataStoreWrite  DataStoreName=temp_1byte  IndexOptions=Index vector (dialog)  Indices=1  OutputSizes=1
  Out : Outport  VectorParamsAs1DForOutWhenUnconnected=off
  wires:
  MCP_RESET/1 -> SPI driver/1
  In/1 -> Out/1
  SPI driver/1 -> Temporary buffer/1

== system Currentreqtest/CANbegin - WARNING, CONTAINS HARDCODED VALUES/setup/setCANRxBuffer ==
  note: RXB0
  note: RXB1
  note: no filter, no mask
  In : Inport
  MCP_RXB0CTRL : Constant  Value=hex2dec('60')  OutDataTypeStr=uint8
  MCP_RXB1CTRL : Constant  Value=hex2dec('70')  OutDataTypeStr=uint8
  MCP_RXB_RX_MASK : Constant  Value=hex2dec('60')  OutDataTypeStr=uint8
  mcp2515_writeRegister : Subsystem  TreatAsAtomicUnit=on
  mcp2515_writeRegister1 : Subsystem  TreatAsAtomicUnit=on
  Out : Outport  VectorParamsAs1DForOutWhenUnconnected=off
  wires:
  MCP_RXB0CTRL/1 -> mcp2515_writeRegister/2(address)
  MCP_RXB1CTRL/1 -> mcp2515_writeRegister1/2(address)
  MCP_RXB_RX_MASK/1 -> mcp2515_writeRegister1/3(value), mcp2515_writeRegister/3(value)
  In/1 -> mcp2515_writeRegister/1(In)
  mcp2515_writeRegister1/1(Out) -> Out/1
  mcp2515_writeRegister/1(Out) -> mcp2515_writeRegister1/1(In)

== system Currentreqtest/CANbegin - WARNING, CONTAINS HARDCODED VALUES/setup/setCANspeed ==
  In : Inport
  CNF1 : Inport  Port=2
  CNF2 : Inport  Port=3
  CNF3 : Inport  Port=4
  MCP_CNF1 : Constant  Value=hex2dec('2A')  OutDataTypeStr=uint8
  MCP_CNF2 : Constant  Value=hex2dec('29')  OutDataTypeStr=uint8
  MCP_CNF3 : Constant  Value=hex2dec('28')  OutDataTypeStr=uint8
  mcp2515_writeRegister1 : Subsystem  TreatAsAtomicUnit=on
  mcp2515_writeRegister2 : Subsystem  TreatAsAtomicUnit=on
  mcp2515_writeRegister3 : Subsystem  TreatAsAtomicUnit=on
  Out : Outport  VectorParamsAs1DForOutWhenUnconnected=off
  wires:
  MCP_CNF2/1 -> mcp2515_writeRegister2/2(address)
  MCP_CNF3/1 -> mcp2515_writeRegister3/2(address)
  CNF3/1 -> mcp2515_writeRegister3/3(value)
  CNF1/1 -> mcp2515_writeRegister1/3(value)
  MCP_CNF1/1 -> mcp2515_writeRegister1/2(address)
  CNF2/1 -> mcp2515_writeRegister2/3(value)
  In/1 -> mcp2515_writeRegister1/1(In)
  mcp2515_writeRegister1/1(Out) -> mcp2515_writeRegister2/1(In)
  mcp2515_writeRegister2/1(Out) -> mcp2515_writeRegister3/1(In)
  mcp2515_writeRegister3/1(Out) -> Out/1

== system Currentreqtest/CANreceive/readRxBuffer/checkRx1Buffer ==
  RX_STATUS : Inport
  Bitmask_RxB1_Status : simulink/Logic and Bit Operations/Bitwise Operator  logicop=AND  UseBitMask=on  BitMask=bin2dec('10000000')  BitMaskRealWorld=Stored Integer
  MCP_READ_RxB0 : Constant  Value=hex2dec('90')  OutDataTypeStr=uint8
  MCP_READ_RxB1 : Constant  Value=hex2dec('94')  OutDataTypeStr=uint8
  Switch : Switch  Criteria=u2 > Threshold  SaturateOnIntegerOverflow=off  InputSameDT=off
  cmd_read_rx_buff : Outport
  wires:
  Switch/1 -> cmd_read_rx_buff/1
  MCP_READ_RxB1/1 -> Switch/1
  MCP_READ_RxB0/1 -> Switch/3
  Bitmask_RxB1_Status/1 -> Switch/2
  RX_STATUS/1 -> Bitmask_RxB1_Status/1

== system Currentreqtest/CANreceive/readRxBuffer/getDLC ==
  RxBx : Inport
  Bitwise Operator : simulink/Logic and Bit Operations/Bitwise Operator  logicop=AND  UseBitMask=off  NumInputPorts=2  BitMask=bin2dec('11011001')  BitMaskRealWorld=Stored Integer
  MCP_DLC_MASK : Constant  Value=hex2dec('0F')  OutDataTypeStr=uint8
  RxDLC : Selector  IndexMode=Zero-based  InputPortWidth=13  IndexOptions=Index vector (dialog)  Indices=4  OutputSizes=1
  CAN_dlc : Outport
  wires:
  Bitwise Operator/1 -> CAN_dlc/1
  RxBx/1 -> RxDLC/1
  RxDLC/1 -> Bitwise Operator/1
  MCP_DLC_MASK/1 -> Bitwise Operator/2

== system Currentreqtest/CANreceive/readRxBuffer/getData ==
  RxBx : Inport
  RxData : Selector  IndexMode=Zero-based  InputPortWidth=13  IndexOptions=Index vector (dialog)  Indices=[5:12]  OutputSizes=1
  CAN_data : Outport
  wires:
  RxBx/1 -> RxData/1
  RxData/1 -> CAN_data/1

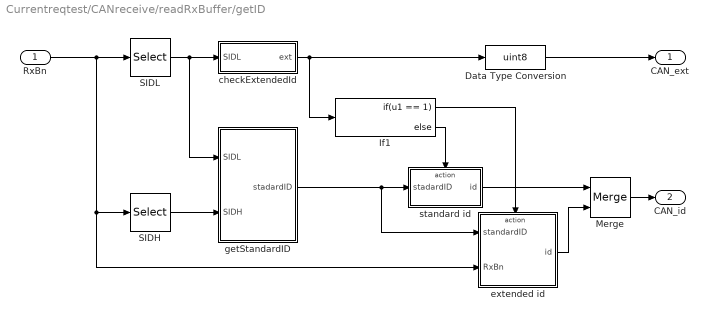
== system Currentreqtest/CANreceive/readRxBuffer/getID ==
  RxBn : Inport
  Data Type Conversion : DataTypeConversion  OutDataTypeStr=uint8  RndMeth=Simplest  SaturateOnIntegerOverflow=off
  If1 : If  IfExpression=u1 == 1
  Merge : Merge
  SIDH : Selector  IndexMode=Zero-based  InputPortWidth=13  IndexOptions=Index vector (dialog)  Indices=0  OutputSizes=1
  SIDL : Selector  IndexMode=Zero-based  InputPortWidth=13  IndexOptions=Index vector (dialog)  Indices=1  OutputSizes=1
  checkExtendedId : Subsystem
  extended id : Subsystem  TreatAsAtomicUnit=on
      settings: RTWSystemCode=Inline
  getStandardID : Subsystem
  standard id : Subsystem  TreatAsAtomicUnit=on
      settings: RTWSystemCode=Inline
  CAN_ext : Outport
  CAN_id : Outport  Port=2
  wires:
  standard id/1(id) -> Merge/1
  extended id/1(id) -> Merge/2
  Merge/1 -> CAN_id/1
  If1/2 -> standard id/Action
  If1/1 -> extended id/Action
  RxBn/1 -> extended id/2(RxBn), SIDH/1, SIDL/1
  getStandardID/1(stadardID) -> standard id/1(stadardID), extended id/1(standardID)
  SIDL/1 -> getStandardID/1(SIDL), checkExtendedId/1(SIDL)
  SIDH/1 -> getStandardID/2(SIDH)
  checkExtendedId/1(ext) -> Data Type Conversion/1, If1/1
  Data Type Conversion/1 -> CAN_ext/1
  ? -> ?

== system Currentreqtest/CANreceive/readRxBuffer/mcp2515_readRxBuffer ==
  In : Inport
  cmd_read_rx_buff : Inport  Port=2
  Constant : Constant  Value=zeros(1,13)  OutDataTypeStr=uint8
  SPI driver : mcp2515lib/CAN application/mcp2515 driver/SPI driver  SystemSampleTime=-1  VariantActivationTime=update diagram  Latency=0  AutoFrameSizeCalculation=off
      settings: SourceProductName=CAN device driver for mcp2515
  Selector1 : Selector  IndexMode=Zero-based  InputPortWidth=14  IndexOptions=Index vector (dialog)  Indices=[1:13]  OutputSizes=1
  Vector Concatenate : Concatenate
  Out : Outport
  RxBn : Outport  Port=2
  wires:
  cmd_read_rx_buff/1 -> Vector Concatenate/1
  Constant/1 -> Vector Concatenate/2
  Vector Concatenate/1 -> SPI driver/1
  SPI driver/1 -> Selector1/1  "SPIout_extd_id"
  Selector1/1 -> RxBn/1
  In/1 -> Out/1

== system Currentreqtest/CAN send LEFT/CANbegin - WARNING, CONTAINS HARDCODED VALUES/setup/changeCANmode(config) ==
  In : Inport
  MCP_CANCTRL : Constant  Value=hex2dec('0F')  OutDataTypeStr=uint8
  MODE_CONFIG : Constant  Value=hex2dec('80')  OutDataTypeStr=uint8
  MODE_MASK : Constant  Value=hex2dec('E0')  OutDataTypeStr=uint8
  mcp2515_modifyRegister : Subsystem  TreatAsAtomicUnit=on
  Out : Outport  VectorParamsAs1DForOutWhenUnconnected=off
  wires:
  MODE_CONFIG/1 -> mcp2515_modifyRegister/4(data)
  MODE_MASK/1 -> mcp2515_modifyRegister/3(mask)
  MCP_CANCTRL/1 -> mcp2515_modifyRegister/2(address)
  In/1 -> mcp2515_modifyRegister/1(In)
  mcp2515_modifyRegister/1(Out) -> Out/1

== system Currentreqtest/CAN send LEFT/CANbegin - WARNING, CONTAINS HARDCODED VALUES/setup/changeCANmode(normal) ==
  In : Inport
  MCP_CANCTRL : Constant  Value=hex2dec('0F')  OutDataTypeStr=uint8
  MODE_MASK : Constant  Value=hex2dec('E0')  OutDataTypeStr=uint8
  MODE_NORMAL : Constant  Value=0  OutDataTypeStr=uint8
  mcp2515_modifyRegister : Subsystem  TreatAsAtomicUnit=on
  Out : Outport  VectorParamsAs1DForOutWhenUnconnected=off
  wires:
  MODE_MASK/1 -> mcp2515_modifyRegister/3(mask)
  MODE_NORMAL/1 -> mcp2515_modifyRegister/4(data)
  MCP_CANCTRL/1 -> mcp2515_modifyRegister/2(address)
  In/1 -> mcp2515_modifyRegister/1(In)
  mcp2515_modifyRegister/1(Out) -> Out/1

== system Currentreqtest/CAN send LEFT/CANbegin - WARNING, CONTAINS HARDCODED VALUES/setup/mcp2515_reset ==
  In : Inport
  MCP_RESET : Constant  Value=hex2dec('C0')  OutDataTypeStr=uint8
  SPI driver : mcp2515lib/CAN application/mcp2515 driver/SPI driver  SystemSampleTime=-1  VariantActivationTime=update diagram  Latency=0  AutoFrameSizeCalculation=off
      settings: SourceProductName=CAN device driver for mcp2515
  Temporary buffer : DataStoreWrite  DataStoreName=temp_1byte  IndexOptions=Index vector (dialog)  Indices=1  OutputSizes=1
  Out : Outport  VectorParamsAs1DForOutWhenUnconnected=off
  wires:
  MCP_RESET/1 -> SPI driver/1
  In/1 -> Out/1
  SPI driver/1 -> Temporary buffer/1
